simulink model "Preliminary_Report_Simulink"  (R2016a)
settings: Solver=VariableStepAuto  StartTime=0.0  StopTime=10  RelTol=1e-3
values from neighbouring files (symbols this model uses):
  f = 8.5*10^-4    (= 0.00085)    [Final_Report_Matlab.m]    (also in Preliminary_Report_Matlab.m)
  J = ((7.1*10^-6)*5.9^2)+(1.4*10^-4)+(2.6*10^-4)    (= 0.000647151)    [Final_Report_Matlab.m]    (also in Preliminary_Report_Matlab.m)
  ke = 2.29*10^-2    (= 0.0229)    [Final_Report_Matlab.m]    (also in Preliminary_Report_Matlab.m)
  kt = 2.29*10^-2    (= 0.0229)    [Final_Report_Matlab.m]    (also in Preliminary_Report_Matlab.m)
  L = 0.66*10^-3    (= 0.00066)    [Final_Report_Matlab.m]    (also in Preliminary_Report_Matlab.m)
  R = 0.71    [Final_Report_Matlab.m]    (also in Preliminary_Report_Matlab.m)
settings Model: Creator=X1  LastModifiedBy=X1

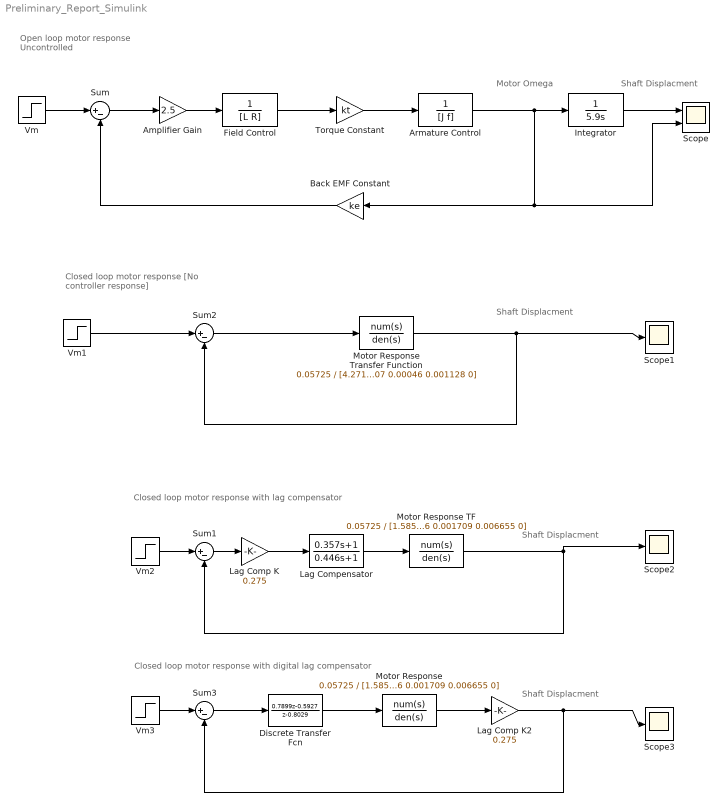
== system Preliminary_Report_Simulink ==
  note: Shaft Displacment
  note: Motor Omega
  note: Open loop motor response
      | Uncontrolled
  note: Shaft Displacment
  note: Closed loop motor response
      | [No controller response]
  note: Shaft Displacment
  note: Closed loop motor response with lag compensator
  note: Shaft Displacment
  note: Closed loop motor response with digital lag compensator
  Amplifier Gain : Gain  Gain=2.5
  Armature Control : TransferFcn  Denominator=[J f]
  Back EMF Constant : Gain  Gain=ke
  Discrete Transfer Fcn : DiscreteTransferFcn  Numerator=[0.7899 -0.5927]  Denominator=[1 -0.8029]  SampleTime=0.1
  Field Control : TransferFcn  Denominator=[L R]
  Integrator : TransferFcn  Denominator=[5.9 0]
  Lag Comp K : Gain  Gain=0.275
  Lag Comp K2 : Gain  Gain=0.275
  Lag Compensator : TransferFcn  Numerator=[0.357 1]  Denominator=[0.446 1]
  Motor Response : TransferFcn  Numerator=0.05725  Denominator=[1.585e-06 0.001709 0.006655 0]
  Motor Response TF : TransferFcn  Numerator=0.05725  Denominator=[1.585e-06 0.001709 0.006655 0]
  Motor Response Transfer Function : TransferFcn  Numerator=0.05725  Denominator=[4.271e-07 0.00046 0.001128 0]
  Scope : Scope  NumInputPorts=2
  Scope1 : Scope
  Scope2 : Scope
  Scope3 : Scope
  Sum{,1..3} (4 alike) : Sum  Inputs=|+-
  Torque Constant : Gain  Gain=kt
  Vm : Step  Time=0  SampleTime=0
  Vm1 : Step  SampleTime=0
  Vm2 : Step  SampleTime=0
  Vm3 : Step  SampleTime=0.1
  wires:
  Torque Constant/1 -> Armature Control/1
  Field Control/1 -> Torque Constant/1
  Back EMF Constant/1 -> Sum/2
  Vm2/1 -> Sum1/1
  Sum1/1 -> Lag Comp K/1
  Lag Comp K/1 -> Lag Compensator/1
  Vm/1 -> Sum/1
  Vm1/1 -> Sum2/1
  Sum2/1 -> Motor Response Transfer Function/1
  Sum/1 -> Amplifier Gain/1
  Integrator/1 -> Scope/1
  Armature Control/1 -> Integrator/1, Scope/2, Back EMF Constant/1
  Motor Response Transfer Function/1 -> Sum2/2, Scope1/1
  Amplifier Gain/1 -> Field Control/1
  Lag Compensator/1 -> Motor Response TF/1
  Motor Response TF/1 -> Sum1/2, Scope2/1
  Vm3/1 -> Sum3/1
  Motor Response/1 -> Lag Comp K2/1
  Lag Comp K2/1 -> Sum3/2, Scope3/1
  Discrete Transfer Fcn/1 -> Motor Response/1
  Sum3/1 -> Discrete Transfer Fcn/1
